simulink model "DOB"  (R2018a)
settings: Solver=VariableStepAuto  StartTime=0.0  StopTime=10  RelTol=1e-3
model workspace (MATLAB code in the model file):
  | Cr=198000;
  | Cf=470000;
  | Mz=1000;
  | lf=3.67;
  | lr=1.93;
  | m=9950;
  | J=5;
  | v=50;
  | nu=1;
  | a0=(Cf*Cr*(lf+lr)^2)+(Cr*lr-Cf*lf)*m*v^2;
  | a1=(Cf*(J+lf^2*m)+Cr*(J+lr^2*m))*v;
  | a2=J*m*v^2;
  | b0=(Cf*Cr*(lf+lr))*v;
  | b1=(Cf*lf)*m*v^2;
  | Kn=(Cf*Cr*(lf+lr)*v)/(Cf*Cr*(lf+lr)^2+(-Cr*lr+Cf*lf)*m*v^2);
libraries: simulink x3
settings Model: Creator=uzeyi  LastModifiedBy=uzeyi

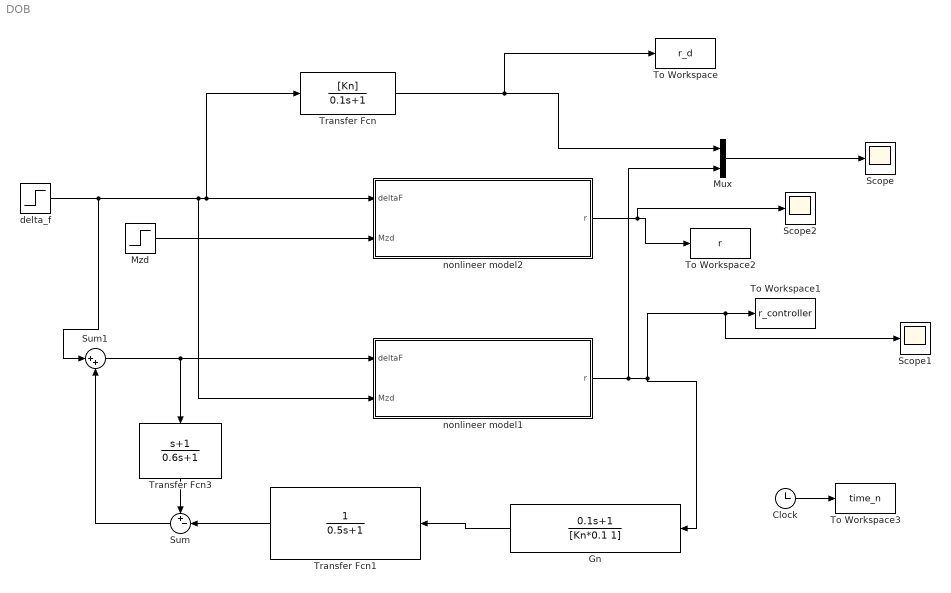
== system DOB ==
  Clock : Clock
  Gn : TransferFcn  Numerator=[0.1 +1]  Denominator=[Kn*0.1 1]
  Mux : Mux  Inputs=2
  Mzd : Step  Time=0  After=1000  SampleTime=0
  Scope : Scope
  Scope1 : Scope
  Scope2 : Scope
  Sum : Sum  Inputs=+-|
  Sum1 : Sum  Inputs=|++
  To Workspace : ToWorkspace  VariableName=r_d  SampleTime=-1
  To Workspace1 : ToWorkspace  VariableName=r_controller  SampleTime=-1
  To Workspace2 : ToWorkspace  VariableName=r  SampleTime=-1
  To Workspace3 : ToWorkspace  VariableName=time_n  SampleTime=-1
  Transfer Fcn : TransferFcn  Numerator=[Kn]  Denominator=[0.1 1]
  Transfer Fcn1 : TransferFcn  Numerator=[ 1]  Denominator=[0.5 1]
  Transfer Fcn3 : TransferFcn  Numerator=[1 1]  Denominator=[0.6 1]
  "delta_f " : Step  Time=0  SampleTime=0
  nonlineer model1 : Subsystem
  nonlineer model2 : Subsystem
  wires:
  "delta_f "/1 -> Sum1/1, Transfer Fcn/1, nonlineer model2/1(deltaF), nonlineer model1/2(Mzd)
  nonlineer model1/1(r) -> Mux/2, Scope1/1, To Workspace1/1, Gn/1
  Mzd/1 -> nonlineer model2/2(Mzd)
  Transfer Fcn1/1 -> Sum/2
  Sum1/1 -> nonlineer model1/1(deltaF), Transfer Fcn3/1
  Transfer Fcn3/1 -> Sum/1
  Sum/1 -> Sum1/2
  Gn/1 -> Transfer Fcn1/1
  Transfer Fcn/1 -> To Workspace/1, Mux/1
  Mux/1 -> Scope/1
  nonlineer model2/1(r) -> Scope2/1, To Workspace2/1
  Clock/1 -> To Workspace3/1

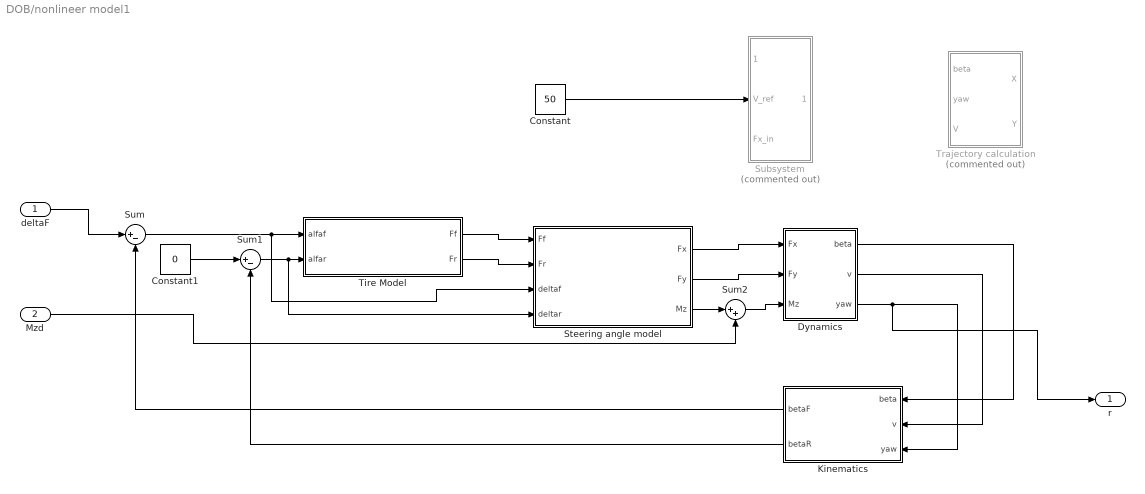
== system DOB/nonlineer model1 ==
  deltaF : Inport
  Mzd : Inport  Port=2
  Constant : Constant  Value=50
  Constant1 : Constant  Value=0
  Dynamics : Subsystem
  "Kinematics\t\t" : Subsystem
  Steering angle model : Subsystem
  Subsystem : Subsystem  Commented=on
  Sum : Sum  Inputs=|+-
  Sum1 : Sum  Inputs=|+-
  Sum2 : Sum  Inputs=|++
  Tire Model : Subsystem
  Trajectory calculation : Subsystem  Commented=on
  r : Outport
  wires:
  Dynamics/2(v) -> "Kinematics\t\t"/2(v)
  Dynamics/3(yaw) -> r/1, "Kinematics\t\t"/3(yaw)
  Steering angle model/2(Fy) -> Dynamics/2(Fy)
  Tire Model/2(Fr) -> Steering angle model/2("Fr ")
  Tire Model/1(Ff) -> Steering angle model/1(Ff)
  Dynamics/1(beta) -> "Kinematics\t\t"/1(beta)
  "Kinematics\t\t"/1(betaF) -> Sum/2
  Sum/1 -> Steering angle model/3("deltaf "), Tire Model/1(alfaf)
  deltaF/1 -> Sum/1
  "Kinematics\t\t"/2(betaR) -> Sum1/2
  Constant1/1 -> Sum1/1
  Sum1/1 -> Steering angle model/4(deltar), Tire Model/2(alfar)
  Constant/1 -> Subsystem/2(V_ref)
  Steering angle model/3(Mz) -> Sum2/1
  Mzd/1 -> Sum2/2
  Sum2/1 -> Dynamics/3(Mz)
  Steering angle model/1(Fx) -> Dynamics/1(Fx)

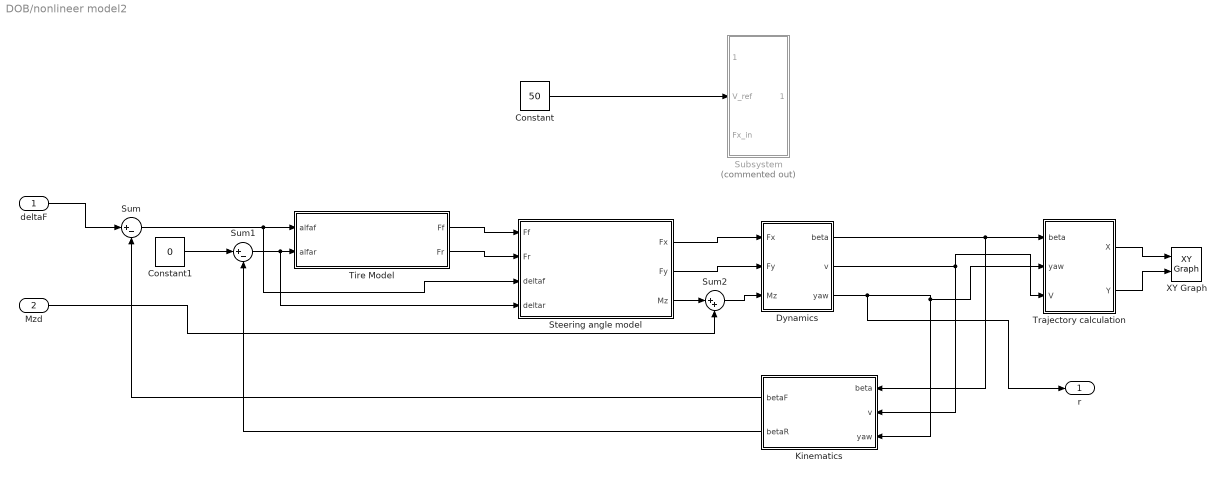
== system DOB/nonlineer model2 ==
  deltaF : Inport
  Mzd : Inport  Port=2
  Constant : Constant  Value=50
  Constant1 : Constant  Value=0
  Dynamics : Subsystem
  "Kinematics\t\t" : Subsystem
  Steering angle model : Subsystem
  Subsystem : Subsystem  Commented=on
  Sum : Sum  Inputs=|+-
  Sum1 : Sum  Inputs=|+-
  Sum2 : Sum  Inputs=|++
  Tire Model : Subsystem
  Trajectory calculation : Subsystem
  XY Graph : simulink/Sinks/XY Graph  xmin=-1  xmax=1  ymin=-1  ymax=1  st=-1
  r : Outport
  wires:
  Dynamics/2(v) -> Trajectory calculation/3(V), "Kinematics\t\t"/2(v)
  Dynamics/3(yaw) -> r/1, Trajectory calculation/2(yaw), "Kinematics\t\t"/3(yaw)
  Steering angle model/2(Fy) -> Dynamics/2(Fy)
  Tire Model/2(Fr) -> Steering angle model/2("Fr ")
  Tire Model/1(Ff) -> Steering angle model/1(Ff)
  Dynamics/1(beta) -> Trajectory calculation/1(beta), "Kinematics\t\t"/1(beta)
  "Kinematics\t\t"/1(betaF) -> Sum/2
  Sum/1 -> Steering angle model/3("deltaf "), Tire Model/1(alfaf)
  deltaF/1 -> Sum/1
  "Kinematics\t\t"/2(betaR) -> Sum1/2
  Constant1/1 -> Sum1/1
  Sum1/1 -> Steering angle model/4(deltar), Tire Model/2(alfar)
  Constant/1 -> Subsystem/2(V_ref)
  Steering angle model/3(Mz) -> Sum2/1
  Mzd/1 -> Sum2/2
  Sum2/1 -> Dynamics/3(Mz)
  Steering angle model/1(Fx) -> Dynamics/1(Fx)
  Trajectory calculation/2(Y) -> XY Graph/2
  Trajectory calculation/1(X) -> XY Graph/1

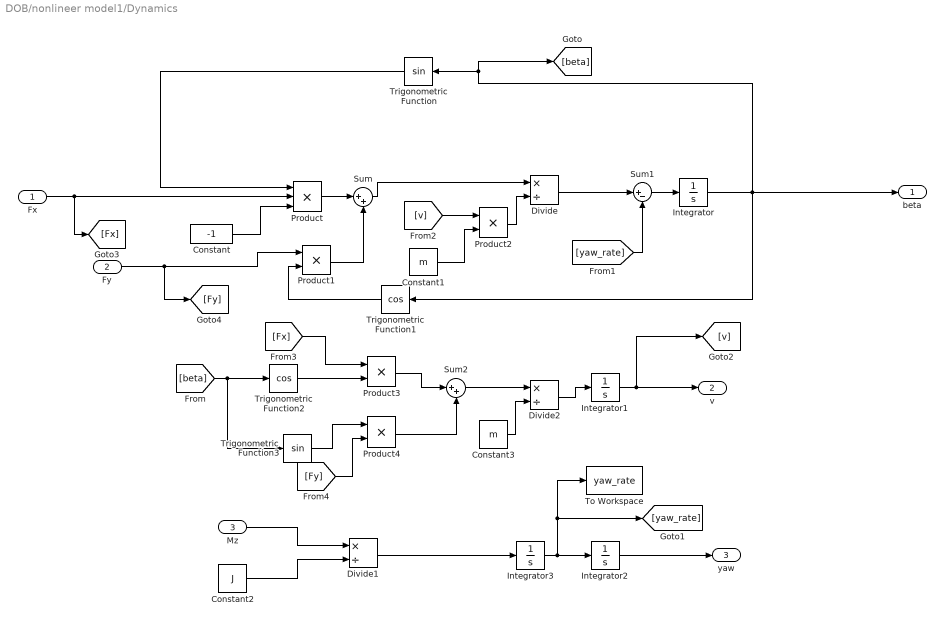
== system DOB/nonlineer model1/Dynamics ==
  Fx : Inport
  Fy : Inport  Port=2
  Mz : Inport  Port=3
  Constant : Constant  Value=-1
  Constant1 : Constant  Value=m
  Constant2 : Constant  Value=J
  Constant3 : Constant  Value=m
  Divide : Product  Inputs=*/
  Divide1 : Product  Inputs=*/
  Divide2 : Product  Inputs=*/
  Integrator : Integrator
  Integrator1 : Integrator  InitialCondition=1
  Integrator2 : Integrator
  Integrator3 : Integrator
  Product : Product  Inputs=3
  Product{1..4} (4 alike) : Product
  Sum : Sum  Inputs=|++
  Sum1 : Sum  Inputs=|+-
  Sum2 : Sum  Inputs=|++
  To Workspace : ToWorkspace  VariableName=yaw_rate  SampleTime=-1
  Trigonometric Function : Trigonometry
  Trigonometric Function1 : Trigonometry  Operator=cos
  Trigonometric Function2 : Trigonometry  Operator=cos
  Trigonometric Function3 : Trigonometry
  beta : Outport
  v : Outport  Port=2
  yaw : Outport  Port=3
  wires:
  Integrator/1 -> Trigonometric Function1/1, [beta], Trigonometric Function/1, beta/1
  Fx/1 -> [Fx], Product/2
  Constant/1 -> Product/3
  Trigonometric Function/1 -> Product/1
  Product/1 -> Sum/1
  Trigonometric Function1/1 -> Product1/2
  Fy/1 -> [Fy], Product1/1
  Product1/1 -> Sum/2
  Sum/1 -> Divide/1
  Integrator1/1 -> [v], v/1
  Integrator2/1 -> yaw/1
  Constant1/1 -> Product2/2
  [v] -> Product2/1
  Product2/1 -> Divide/2
  Sum1/1 -> Integrator/1
  Divide/1 -> Sum1/1
  [yaw_rate] -> Sum1/2
  Integrator3/1 -> [yaw_rate], To Workspace/1, Integrator2/1
  Constant2/1 -> Divide1/2
  Mz/1 -> Divide1/1
  Divide1/1 -> Integrator3/1
  [beta] -> Trigonometric Function3/1, Trigonometric Function2/1
  Trigonometric Function2/1 -> Product3/2
  [Fx] -> Product3/1
  Trigonometric Function3/1 -> Product4/1
  [Fy] -> Product4/2
  Product3/1 -> Sum2/1
  Product4/1 -> Sum2/2
  Sum2/1 -> Divide2/1
  Divide2/1 -> Integrator1/1
  Constant3/1 -> Divide2/2

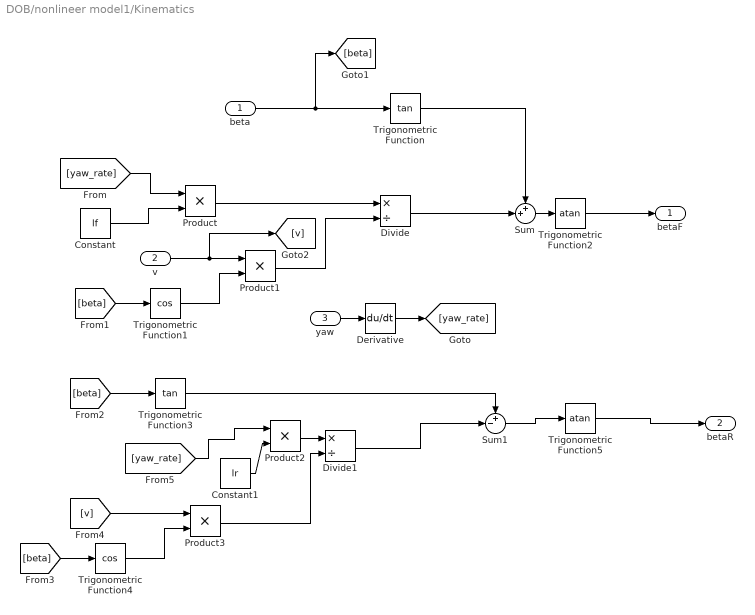
== system DOB/nonlineer model1/Kinematics		 ==
  beta : Inport
  v : Inport  Port=2
  yaw : Inport  Port=3
  Constant : Constant  Value=lf
  Constant1 : Constant  Value=lr
  Derivative : Derivative
  Divide : Product  Inputs=*/
  Divide1 : Product  Inputs=*/
  Product{,1..3} (4 alike) : Product
  Sum : Sum  Inputs=++|
  Sum1 : Sum  Inputs=+-|
  Trigonometric Function : Trigonometry  Operator=tan
  Trigonometric Function1 : Trigonometry  Operator=cos
  Trigonometric Function2 : Trigonometry  Operator=atan
  Trigonometric Function3 : Trigonometry  Operator=tan
  Trigonometric Function4 : Trigonometry  Operator=cos
  Trigonometric Function5 : Trigonometry  Operator=atan
  betaF : Outport
  betaR : Outport  Port=2
  wires:
  beta/1 -> [beta], Trigonometric Function/1
  yaw/1 -> Derivative/1
  [yaw_rate] -> Product/1
  Constant/1 -> Product/2
  Product/1 -> Divide/1
  v/1 -> [v], Product1/1
  [beta] -> Trigonometric Function1/1
  Product1/1 -> Divide/2
  Trigonometric Function1/1 -> Product1/2
  Divide/1 -> Sum/2
  Trigonometric Function/1 -> Sum/1
  Sum/1 -> Trigonometric Function2/1
  Trigonometric Function2/1 -> betaF/1
  Derivative/1 -> [yaw_rate]
  [beta] -> Trigonometric Function3/1
  Trigonometric Function3/1 -> Sum1/1
  Divide1/1 -> Sum1/2
  [beta] -> Trigonometric Function4/1
  Trigonometric Function4/1 -> Product3/2
  Product3/1 -> Divide1/2
  [v] -> Product3/1
  Constant1/1 -> Product2/2
  [yaw_rate] -> Product2/1
  Product2/1 -> Divide1/1
  Sum1/1 -> Trigonometric Function5/1
  Trigonometric Function5/1 -> betaR/1

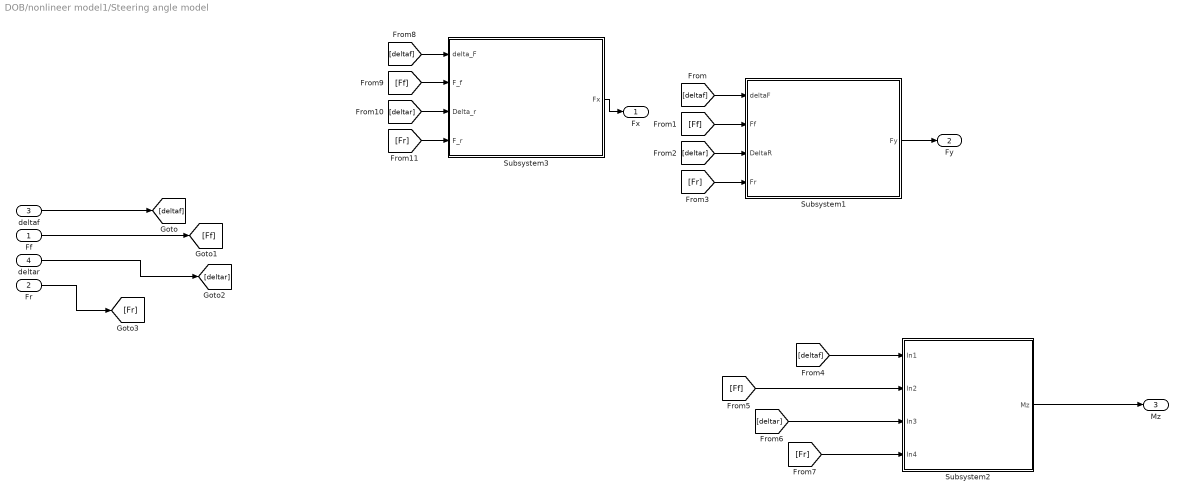
== system DOB/nonlineer model1/Steering angle model ==
  Ff : Inport
  "Fr " : Inport  Port=2
  "deltaf " : Inport  Port=3
  deltar : Inport  Port=4
  Subsystem1 : Subsystem
  Subsystem2 : Subsystem
  Subsystem3 : Subsystem
  Fx : Outport
  Fy : Outport  Port=2
  Mz : Outport  Port=3
  wires:
  "deltaf "/1 -> [deltaf]
  Ff/1 -> [Ff]
  "Fr "/1 -> [Fr]
  deltar/1 -> [deltar]
  [deltaf] -> Subsystem1/1("deltaF ")
  [Ff] -> Subsystem1/2(Ff)
  [deltar] -> Subsystem1/3(DeltaR)
  [Fr] -> Subsystem1/4(Fr)
  Subsystem1/1(Fy) -> Fy/1
  [deltaf] -> Subsystem2/1(In1)
  [Ff] -> Subsystem2/2(In2)
  [deltar] -> Subsystem2/3(In3)
  [Fr] -> Subsystem2/4(In4)
  Subsystem2/1(Mz) -> Mz/1
  [deltaf] -> Subsystem3/1(delta_F)
  [Ff] -> Subsystem3/2(F_f)
  [deltar] -> Subsystem3/3(Delta_r)
  [Fr] -> Subsystem3/4(F_r)
  Subsystem3/1(Fx) -> Fx/1

== system DOB/nonlineer model1/Subsystem ==
  "V_mesaured " : Inport
  V_ref : Inport  Port=2
  Fx_in : Inport  Port=3
  PID Controller : simulink/Continuous/PID Controller  Controller=PID  TimeDomain=Continuous-time  SampleTime=-1  IntegratorMethod=Forward Euler  FilterMethod=Forward Euler  Form=Parallel  UseFilter=on  ControllerParametersSource=internal  P=488771.135263171  I=3246206.54450336  D=-1108.70203647941  N=35.5782515442806  InitialConditionSource=internal  InitialConditionForIntegrator=0  InitialConditionForFilter=0  ExternalReset=none  LimitOutput=off  UpperSaturationLimit=inf  LowerSaturationLimit=-inf  LinearizeAsGain=on  AntiWindupMode=none  Kb=1  TrackingMode=off  Kt=1  PParamMin=[]  PParamMax=[]  IParamMin=[]  IParamMax=[]  DParamMin=[]  DParamMax=[]  NParamMin=[]  NParamMax=[]  KbParamMin=[]  KbParamMax=[]  KtParamMin=[]  KtParamMax=[]  POutMin=[]  POutMax=[]  IOutMin=[]  IOutMax=[]  DOutMin=[]  DOutMax=[]  NOutMin=[]  NOutMax=[]  KbOutMin=[]  KbOutMax=[]  KtOutMin=[]  KtOutMax=[]  IntegratorOutMin=[]  IntegratorOutMax=[]  FilterOutMin=[]  FilterOutMax=[]  SumOutMin=[]  SumOutMax=[]  SumI1OutMin=[]  SumI1OutMax=[]  SumI2OutMin=[]  SumI2OutMax=[]  SumI3OutMin=[]  SumI3OutMax=[]  SumDOutMin=[]  SumDOutMax=[]  SaturationOutMin=[]  SaturationOutMax=[]  IntegratorContinuousStateAttributes=''  IntegratorStateMustResolveToSignalObject=off  IntegratorRTWStateStorageClass=Auto  FilterContinuousStateAttributes=''  FilterStateMustResolveToSignalObject=off  FilterRTWStateStorageClass=Auto  DifferentiatorICPrevScaledInput=0  DifferentiatorOutMin=[]  DifferentiatorOutMax=[]  FilterDiffOutCoefMin=[]  FilterDiffOutCoefMax=[]  SumDenOutMin=[]  SumDenOutMax=[]  SumNumOutMin=[]  SumNumOutMax=[]  ReciprocalOutMin=[]  ReciprocalOutMax=[]  DivideOutMin=[]  DivideOutMax=[]  TunerSelectOption=Transfer Function Based (PID Tuner App)
  Scope : Scope
  Sum : Sum  Inputs=|+-
  Sum1 : Sum  Inputs=|++
  Fx_out : Outport
  wires:
  V_ref/1 -> Sum/1
  "V_mesaured "/1 -> Sum/2
  Sum/1 -> Scope/1, PID Controller/1
  PID Controller/1 -> Sum1/1
  Sum1/1 -> Fx_out/1
  Fx_in/1 -> Sum1/2

== system DOB/nonlineer model1/Tire Model ==
  alfaf : Inport
  alfar : Inport  Port=2
  Constant1 : Constant  Value=Cf
  Constant2 : Constant  Value=Cr
  Constant3 : Constant  Value=nu
  Product : Product  Inputs=3
  Product1 : Product  Inputs=3
  Ff : Outport
  Fr : Outport  Port=2
  wires:
  alfar/1 -> Product/1
  Constant2/1 -> Product/2
  Constant1/1 -> Product1/2
  alfaf/1 -> Product1/1
  Product1/1 -> Ff/1
  Product/1 -> Fr/1
  Constant3/1 -> Product/3, Product1/3

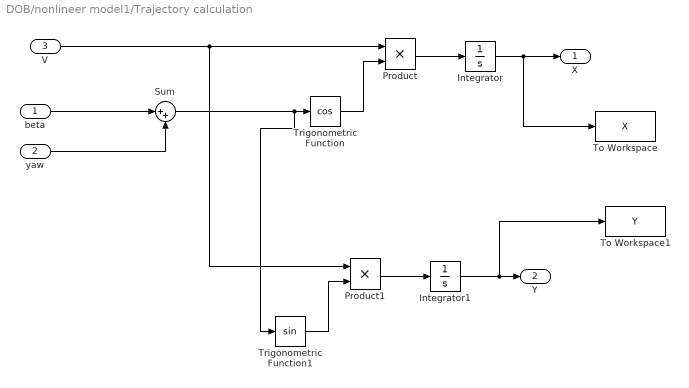
== system DOB/nonlineer model1/Trajectory calculation ==
  beta : Inport
  yaw : Inport  Port=2
  V : Inport  Port=3
  Integrator : Integrator
  Integrator1 : Integrator
  Product : Product
  Product1 : Product
  Sum : Sum  Inputs=|++
  To Workspace : ToWorkspace  VariableName=X  SampleTime=-1
  To Workspace1 : ToWorkspace  VariableName=Y  SampleTime=-1
  Trigonometric Function : Trigonometry  Operator=cos
  Trigonometric Function1 : Trigonometry
  X : Outport
  Y : Outport  Port=2
  wires:
  V/1 -> Product1/1, Product/1
  beta/1 -> Sum/1
  Sum/1 -> Trigonometric Function1/1, Trigonometric Function/1
  Trigonometric Function/1 -> Product/2
  Product/1 -> Integrator/1
  Trigonometric Function1/1 -> Product1/2
  Product1/1 -> Integrator1/1
  Integrator1/1 -> To Workspace1/1, Y/1
  Integrator/1 -> To Workspace/1, X/1
  yaw/1 -> Sum/2

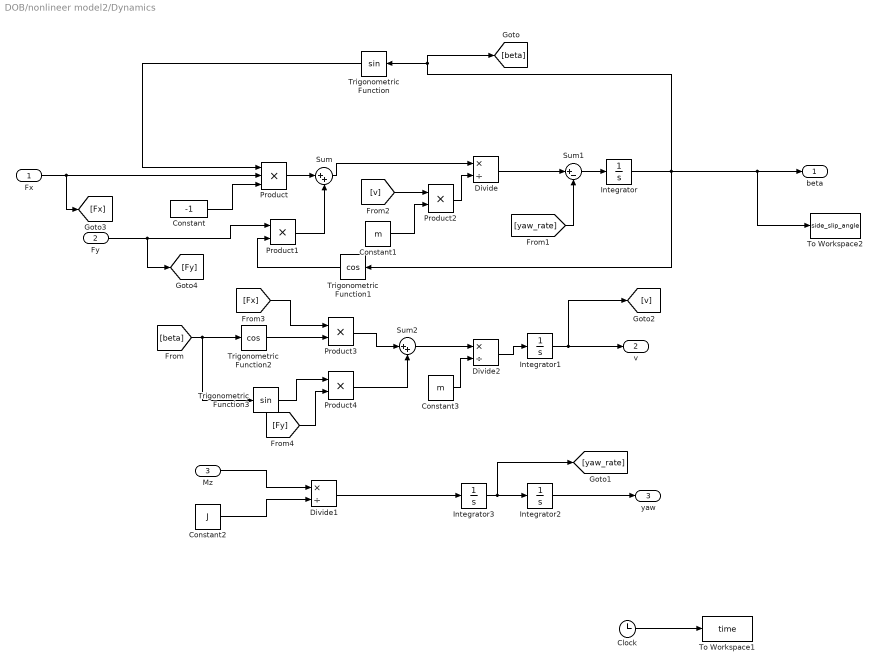
== system DOB/nonlineer model2/Dynamics ==
  Fx : Inport
  Fy : Inport  Port=2
  Mz : Inport  Port=3
  Clock : Clock
  Constant : Constant  Value=-1
  Constant1 : Constant  Value=m
  Constant2 : Constant  Value=J
  Constant3 : Constant  Value=m
  Divide : Product  Inputs=*/
  Divide1 : Product  Inputs=*/
  Divide2 : Product  Inputs=*/
  Integrator : Integrator
  Integrator1 : Integrator  InitialCondition=1
  Integrator2 : Integrator
  Integrator3 : Integrator
  Product : Product  Inputs=3
  Product{1..4} (4 alike) : Product
  Sum : Sum  Inputs=|++
  Sum1 : Sum  Inputs=|+-
  Sum2 : Sum  Inputs=|++
  To Workspace1 : ToWorkspace  VariableName=time  SampleTime=-1
  To Workspace2 : ToWorkspace  VariableName=side_slip_angle  SampleTime=-1
  Trigonometric Function : Trigonometry
  Trigonometric Function1 : Trigonometry  Operator=cos
  Trigonometric Function2 : Trigonometry  Operator=cos
  Trigonometric Function3 : Trigonometry
  beta : Outport
  v : Outport  Port=2
  yaw : Outport  Port=3
  wires:
  Integrator/1 -> Trigonometric Function1/1, [beta], Trigonometric Function/1, To Workspace2/1, beta/1
  Fx/1 -> [Fx], Product/2
  Constant/1 -> Product/3
  Trigonometric Function/1 -> Product/1
  Product/1 -> Sum/1
  Trigonometric Function1/1 -> Product1/2
  Fy/1 -> [Fy], Product1/1
  Product1/1 -> Sum/2
  Sum/1 -> Divide/1
  Integrator1/1 -> [v], v/1
  Integrator2/1 -> yaw/1
  Constant1/1 -> Product2/2
  [v] -> Product2/1
  Product2/1 -> Divide/2
  Sum1/1 -> Integrator/1
  Divide/1 -> Sum1/1
  [yaw_rate] -> Sum1/2
  Integrator3/1 -> [yaw_rate], Integrator2/1
  Constant2/1 -> Divide1/2
  Mz/1 -> Divide1/1
  Divide1/1 -> Integrator3/1
  [beta] -> Trigonometric Function3/1, Trigonometric Function2/1
  Trigonometric Function2/1 -> Product3/2
  [Fx] -> Product3/1
  Trigonometric Function3/1 -> Product4/1
  [Fy] -> Product4/2
  Product3/1 -> Sum2/1
  Product4/1 -> Sum2/2
  Sum2/1 -> Divide2/1
  Divide2/1 -> Integrator1/1
  Constant3/1 -> Divide2/2
  Clock/1 -> To Workspace1/1

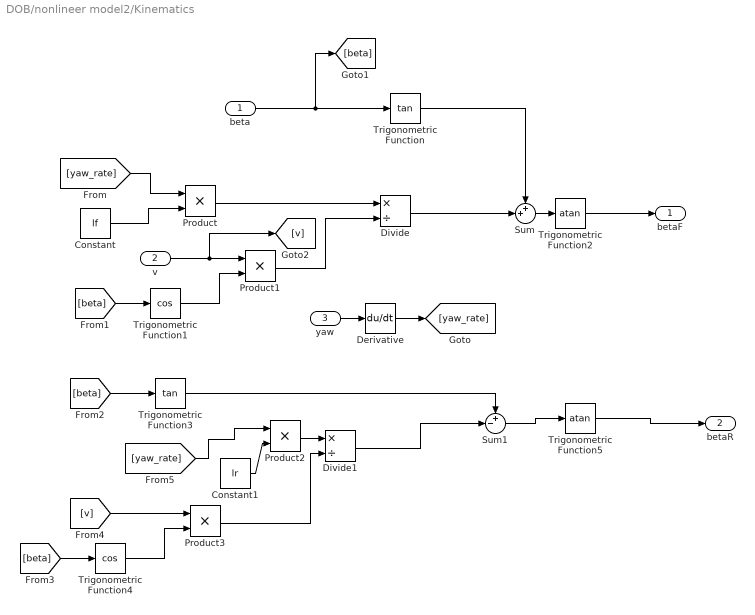
== system DOB/nonlineer model2/Kinematics		 ==
  beta : Inport
  v : Inport  Port=2
  yaw : Inport  Port=3
  Constant : Constant  Value=lf
  Constant1 : Constant  Value=lr
  Derivative : Derivative
  Divide : Product  Inputs=*/
  Divide1 : Product  Inputs=*/
  Product{,1..3} (4 alike) : Product
  Sum : Sum  Inputs=++|
  Sum1 : Sum  Inputs=+-|
  Trigonometric Function : Trigonometry  Operator=tan
  Trigonometric Function1 : Trigonometry  Operator=cos
  Trigonometric Function2 : Trigonometry  Operator=atan
  Trigonometric Function3 : Trigonometry  Operator=tan
  Trigonometric Function4 : Trigonometry  Operator=cos
  Trigonometric Function5 : Trigonometry  Operator=atan
  betaF : Outport
  betaR : Outport  Port=2
  wires:
  beta/1 -> [beta], Trigonometric Function/1
  yaw/1 -> Derivative/1
  [yaw_rate] -> Product/1
  Constant/1 -> Product/2
  Product/1 -> Divide/1
  v/1 -> [v], Product1/1
  [beta] -> Trigonometric Function1/1
  Product1/1 -> Divide/2
  Trigonometric Function1/1 -> Product1/2
  Divide/1 -> Sum/2
  Trigonometric Function/1 -> Sum/1
  Sum/1 -> Trigonometric Function2/1
  Trigonometric Function2/1 -> betaF/1
  Derivative/1 -> [yaw_rate]
  [beta] -> Trigonometric Function3/1
  Trigonometric Function3/1 -> Sum1/1
  Divide1/1 -> Sum1/2
  [beta] -> Trigonometric Function4/1
  Trigonometric Function4/1 -> Product3/2
  Product3/1 -> Divide1/2
  [v] -> Product3/1
  Constant1/1 -> Product2/2
  [yaw_rate] -> Product2/1
  Product2/1 -> Divide1/1
  Sum1/1 -> Trigonometric Function5/1
  Trigonometric Function5/1 -> betaR/1

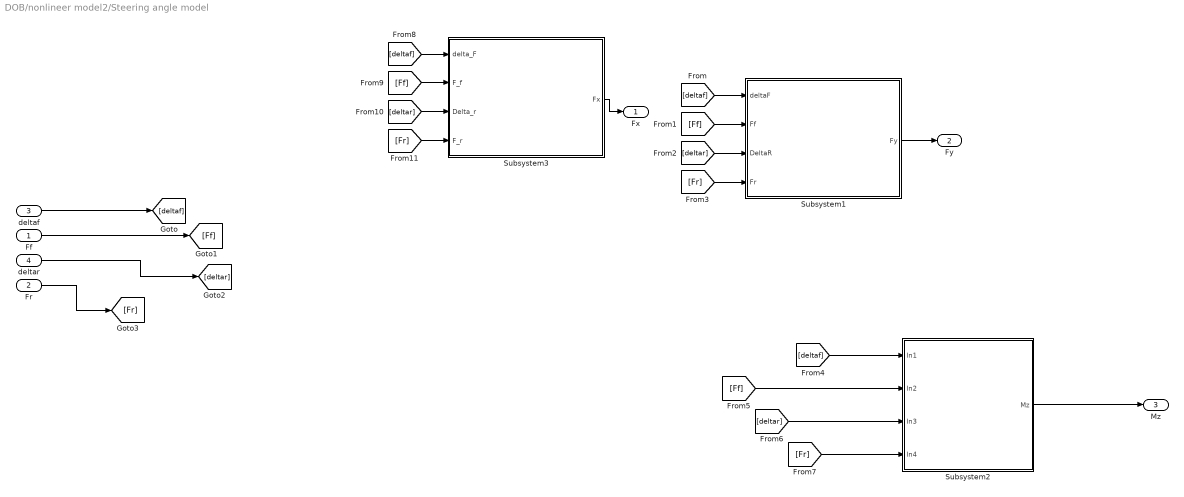
== system DOB/nonlineer model2/Steering angle model ==
  Ff : Inport
  "Fr " : Inport  Port=2
  "deltaf " : Inport  Port=3
  deltar : Inport  Port=4
  Subsystem1 : Subsystem
  Subsystem2 : Subsystem
  Subsystem3 : Subsystem
  Fx : Outport
  Fy : Outport  Port=2
  Mz : Outport  Port=3
  wires:
  "deltaf "/1 -> [deltaf]
  Ff/1 -> [Ff]
  "Fr "/1 -> [Fr]
  deltar/1 -> [deltar]
  [deltaf] -> Subsystem1/1("deltaF ")
  [Ff] -> Subsystem1/2(Ff)
  [deltar] -> Subsystem1/3(DeltaR)
  [Fr] -> Subsystem1/4(Fr)
  Subsystem1/1(Fy) -> Fy/1
  [deltaf] -> Subsystem2/1(In1)
  [Ff] -> Subsystem2/2(In2)
  [deltar] -> Subsystem2/3(In3)
  [Fr] -> Subsystem2/4(In4)
  Subsystem2/1(Mz) -> Mz/1
  [deltaf] -> Subsystem3/1(delta_F)
  [Ff] -> Subsystem3/2(F_f)
  [deltar] -> Subsystem3/3(Delta_r)
  [Fr] -> Subsystem3/4(F_r)
  Subsystem3/1(Fx) -> Fx/1

== system DOB/nonlineer model2/Subsystem ==
  "V_mesaured " : Inport
  V_ref : Inport  Port=2
  Fx_in : Inport  Port=3
  PID Controller : simulink/Continuous/PID Controller  Controller=PID  TimeDomain=Continuous-time  SampleTime=-1  IntegratorMethod=Forward Euler  FilterMethod=Forward Euler  Form=Parallel  UseFilter=on  ControllerParametersSource=internal  P=488771.135263171  I=3246206.54450336  D=-1108.70203647941  N=35.5782515442806  InitialConditionSource=internal  InitialConditionForIntegrator=0  InitialConditionForFilter=0  ExternalReset=none  LimitOutput=off  UpperSaturationLimit=inf  LowerSaturationLimit=-inf  LinearizeAsGain=on  AntiWindupMode=none  Kb=1  TrackingMode=off  Kt=1  PParamMin=[]  PParamMax=[]  IParamMin=[]  IParamMax=[]  DParamMin=[]  DParamMax=[]  NParamMin=[]  NParamMax=[]  KbParamMin=[]  KbParamMax=[]  KtParamMin=[]  KtParamMax=[]  POutMin=[]  POutMax=[]  IOutMin=[]  IOutMax=[]  DOutMin=[]  DOutMax=[]  NOutMin=[]  NOutMax=[]  KbOutMin=[]  KbOutMax=[]  KtOutMin=[]  KtOutMax=[]  IntegratorOutMin=[]  IntegratorOutMax=[]  FilterOutMin=[]  FilterOutMax=[]  SumOutMin=[]  SumOutMax=[]  SumI1OutMin=[]  SumI1OutMax=[]  SumI2OutMin=[]  SumI2OutMax=[]  SumI3OutMin=[]  SumI3OutMax=[]  SumDOutMin=[]  SumDOutMax=[]  SaturationOutMin=[]  SaturationOutMax=[]  IntegratorContinuousStateAttributes=''  IntegratorStateMustResolveToSignalObject=off  IntegratorRTWStateStorageClass=Auto  FilterContinuousStateAttributes=''  FilterStateMustResolveToSignalObject=off  FilterRTWStateStorageClass=Auto  DifferentiatorICPrevScaledInput=0  DifferentiatorOutMin=[]  DifferentiatorOutMax=[]  FilterDiffOutCoefMin=[]  FilterDiffOutCoefMax=[]  SumDenOutMin=[]  SumDenOutMax=[]  SumNumOutMin=[]  SumNumOutMax=[]  ReciprocalOutMin=[]  ReciprocalOutMax=[]  DivideOutMin=[]  DivideOutMax=[]  TunerSelectOption=Transfer Function Based (PID Tuner App)
  Scope : Scope
  Sum : Sum  Inputs=|+-
  Sum1 : Sum  Inputs=|++
  Fx_out : Outport
  wires:
  V_ref/1 -> Sum/1
  "V_mesaured "/1 -> Sum/2
  Sum/1 -> Scope/1, PID Controller/1
  PID Controller/1 -> Sum1/1
  Sum1/1 -> Fx_out/1
  Fx_in/1 -> Sum1/2

== system DOB/nonlineer model2/Tire Model ==
  alfaf : Inport
  alfar : Inport  Port=2
  Constant1 : Constant  Value=Cf
  Constant2 : Constant  Value=Cr
  Constant3 : Constant  Value=nu
  Product : Product  Inputs=3
  Product1 : Product  Inputs=3
  Ff : Outport
  Fr : Outport  Port=2
  wires:
  alfar/1 -> Product/1
  Constant2/1 -> Product/2
  Constant1/1 -> Product1/2
  alfaf/1 -> Product1/1
  Product1/1 -> Ff/1
  Product/1 -> Fr/1
  Constant3/1 -> Product/3, Product1/3

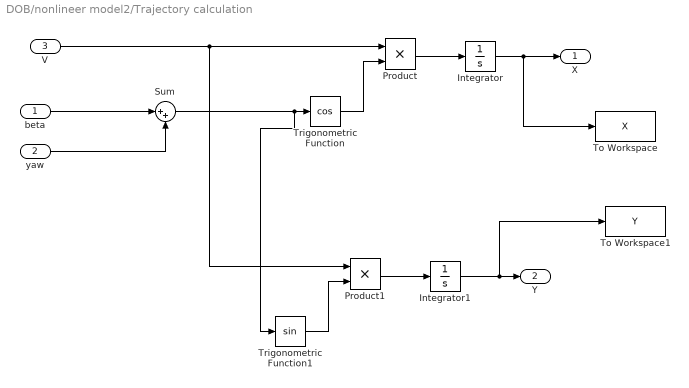
== system DOB/nonlineer model2/Trajectory calculation ==
  beta : Inport
  yaw : Inport  Port=2
  V : Inport  Port=3
  Integrator : Integrator
  Integrator1 : Integrator
  Product : Product
  Product1 : Product
  Sum : Sum  Inputs=|++
  To Workspace : ToWorkspace  VariableName=X  SampleTime=-1
  To Workspace1 : ToWorkspace  VariableName=Y  SampleTime=-1
  Trigonometric Function : Trigonometry  Operator=cos
  Trigonometric Function1 : Trigonometry
  X : Outport
  Y : Outport  Port=2
  wires:
  V/1 -> Product1/1, Product/1
  beta/1 -> Sum/1
  Sum/1 -> Trigonometric Function1/1, Trigonometric Function/1
  Trigonometric Function/1 -> Product/2
  Product/1 -> Integrator/1
  Trigonometric Function1/1 -> Product1/2
  Product1/1 -> Integrator1/1
  Integrator1/1 -> To Workspace1/1, Y/1
  Integrator/1 -> To Workspace/1, X/1
  yaw/1 -> Sum/2

== system DOB/nonlineer model1/Steering angle model/Subsystem1 ==
  "deltaF " : Inport
  Ff : Inport  Port=2
  DeltaR : Inport  Port=3
  Fr : Inport  Port=4
  Product3 : Product
  Product4 : Product
  Sum1 : Sum  Inputs=|++
  Trigonometric Function2 : Trigonometry  Operator=cos
  Trigonometric Function3 : Trigonometry  Operator=cos
  Fy : Outport
  wires:
  Product3/1 -> Sum1/1
  Product4/1 -> Sum1/2
  DeltaR/1 -> Trigonometric Function3/1
  Sum1/1 -> Fy/1
  Trigonometric Function2/1 -> Product3/1
  Trigonometric Function3/1 -> Product4/1
  Fr/1 -> Product4/2
  "deltaF "/1 -> Trigonometric Function2/1
  Ff/1 -> Product3/2

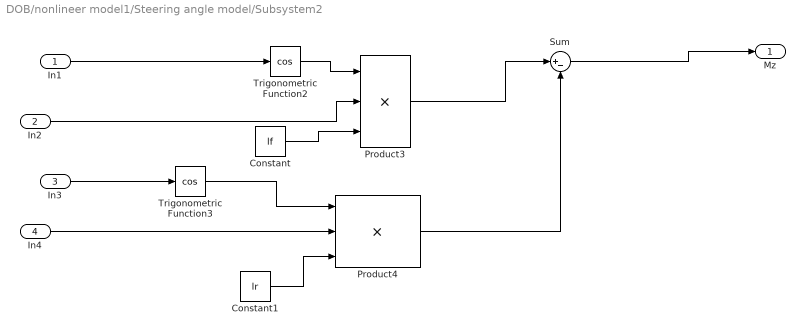
== system DOB/nonlineer model1/Steering angle model/Subsystem2 ==
  In1 : Inport
  In2 : Inport  Port=2
  In3 : Inport  Port=3
  In4 : Inport  Port=4
  Constant : Constant  Value=lf
  Constant1 : Constant  Value=lr
  Product3 : Product  Inputs=3
  Product4 : Product  Inputs=3
  Sum : Sum  Inputs=|+-
  Trigonometric Function2 : Trigonometry  Operator=cos
  Trigonometric Function3 : Trigonometry  Operator=cos
  Mz : Outport
  wires:
  Constant1/1 -> Product4/3
  Constant/1 -> Product3/3
  In3/1 -> Trigonometric Function3/1
  Product3/1 -> Sum/1
  Product4/1 -> Sum/2
  In2/1 -> Product3/2
  In4/1 -> Product4/2
  In1/1 -> Trigonometric Function2/1
  Trigonometric Function2/1 -> Product3/1
  Trigonometric Function3/1 -> Product4/1
  Sum/1 -> Mz/1

== system DOB/nonlineer model1/Steering angle model/Subsystem3 ==
  delta_F : Inport
  F_f : Inport  Port=2
  Delta_r : Inport  Port=3
  F_r : Inport  Port=4
  Constant : Constant
  Product1 : Product
  Product3 : Product
  Product4 : Product
  Sum1 : Sum  Inputs=|++
  Trigonometric Function2 : Trigonometry
  Trigonometric Function3 : Trigonometry
  Fx : Outport
  wires:
  Product3/1 -> Sum1/1
  Product4/1 -> Sum1/2
  Delta_r/1 -> Trigonometric Function3/1
  Trigonometric Function2/1 -> Product3/1
  Trigonometric Function3/1 -> Product4/1
  F_r/1 -> Product4/2
  delta_F/1 -> Trigonometric Function2/1
  F_f/1 -> Product3/2
  Sum1/1 -> Product1/1
  Product1/1 -> Fx/1
  Constant/1 -> Product1/2

== system DOB/nonlineer model2/Steering angle model/Subsystem1 ==
  "deltaF " : Inport
  Ff : Inport  Port=2
  DeltaR : Inport  Port=3
  Fr : Inport  Port=4
  Product3 : Product
  Product4 : Product
  Sum1 : Sum  Inputs=|++
  Trigonometric Function2 : Trigonometry  Operator=cos
  Trigonometric Function3 : Trigonometry  Operator=cos
  Fy : Outport
  wires:
  Product3/1 -> Sum1/1
  Product4/1 -> Sum1/2
  DeltaR/1 -> Trigonometric Function3/1
  Sum1/1 -> Fy/1
  Trigonometric Function2/1 -> Product3/1
  Trigonometric Function3/1 -> Product4/1
  Fr/1 -> Product4/2
  "deltaF "/1 -> Trigonometric Function2/1
  Ff/1 -> Product3/2

== system DOB/nonlineer model2/Steering angle model/Subsystem2 ==
  In1 : Inport
  In2 : Inport  Port=2
  In3 : Inport  Port=3
  In4 : Inport  Port=4
  Constant : Constant  Value=lf
  Constant1 : Constant  Value=lr
  Product3 : Product  Inputs=3
  Product4 : Product  Inputs=3
  Sum : Sum  Inputs=|+-
  Trigonometric Function2 : Trigonometry  Operator=cos
  Trigonometric Function3 : Trigonometry  Operator=cos
  Mz : Outport
  wires:
  Constant1/1 -> Product4/3
  Constant/1 -> Product3/3
  In3/1 -> Trigonometric Function3/1
  Product3/1 -> Sum/1
  Product4/1 -> Sum/2
  In2/1 -> Product3/2
  In4/1 -> Product4/2
  In1/1 -> Trigonometric Function2/1
  Trigonometric Function2/1 -> Product3/1
  Trigonometric Function3/1 -> Product4/1
  Sum/1 -> Mz/1

== system DOB/nonlineer model2/Steering angle model/Subsystem3 ==
  delta_F : Inport
  F_f : Inport  Port=2
  Delta_r : Inport  Port=3
  F_r : Inport  Port=4
  Constant : Constant
  Product1 : Product
  Product3 : Product
  Product4 : Product
  Sum1 : Sum  Inputs=|++
  Trigonometric Function2 : Trigonometry
  Trigonometric Function3 : Trigonometry
  Fx : Outport
  wires:
  Product3/1 -> Sum1/1
  Product4/1 -> Sum1/2
  Delta_r/1 -> Trigonometric Function3/1
  Trigonometric Function2/1 -> Product3/1
  Trigonometric Function3/1 -> Product4/1
  F_r/1 -> Product4/2
  delta_F/1 -> Trigonometric Function2/1
  F_f/1 -> Product3/2
  Sum1/1 -> Product1/1
  Product1/1 -> Fx/1
  Constant/1 -> Product1/2
